simulink model "sim_accelerometersensor1"  (R2020b)
settings: Solver=FixedStepDiscrete  StartTime=0.0  StopTime=60  FixedStep=0.1  RelTol=1e-3  EnableMultiTasking=on
undefined symbols (not defined in the file): DiscIntNeverNeededParam
libraries: frdmk64flib x3, dspstat3 x2
settings Model: ExtModeTrigDuration=5  Creator=luca9  LastModifiedBy=luca9
settings OptimizationCC: EnhancedBackFolding=on  PassReuseOutputArgsAs=Individual arguments  ZeroExternalMemoryAtStartup=off  ZeroInternalMemoryAtStartup=off  MaxStackSize=64  OptimizeBlockOrder=speed  DifferentSizesBufferReuse=on  OptimizationCustomize=off  EfficientTunableParamExpr=on
settings DebuggingCC: ParameterTunabilityLossMsg=error
settings HardwareCC: ProdBitPerPointer=32  ProdBitPerSizeT=32  ProdBitPerPtrDiffT=32  ProdLargestAtomicInteger=Long  ProdLargestAtomicFloat=Double  ProdWordSize=32  ProdHWDeviceType=ARM Compatible->ARM Cortex
settings SFSimCC: MATLABDynamicMemAlloc=off
settings RTWCC: Description=Embedded Coder  SystemTargetFile=ert.tlc  HardwareBoard=NXP FRDM-K64F  TLCOptions="-aInlineSetEventsForThisBaseRateFcn=TLC_FALSE -aSuppressMultiTaskScheduler=TLC_FALSE  -aRateBasedStepFcn=0"  TemplateMakefile=ert_default_tmf  GenerateReport=on  Toolchain=GNU Tools for ARM Embedded Processors
settings CodeAppCC: ForceParamTrailComments=on  IgnoreCustomStorageClasses=off  OperatorAnnotations=on  SimulinkDataObjDesc=on  SFDataObjDesc=on  InsertBlockDesc=on

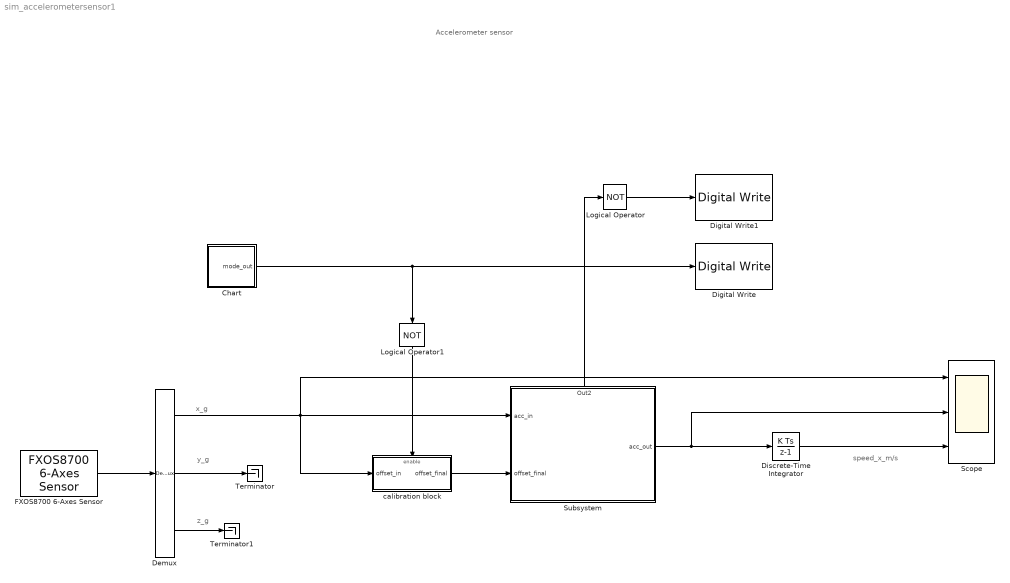
== system sim_accelerometersensor1 ==
  note: Accelerometer sensor
  note: speed_x_m/s
  note: z_g
  note: y_g
  note: x_g
  Chart : Stateflow chart  TreatAsAtomicUnit=on
  Demux : Demux  Outputs=3
  Digital Write : frdmk64flib/Digital Write  Whichpin=GREEN_LED
  Digital Write1 : frdmk64flib/Digital Write  Whichpin=RED_LED
  Discrete-Time Integrator : DiscreteIntegrator  SampleTime=-1  ICPrevOutput=DiscIntNeverNeededParam  ICPrevScaledInput=DiscIntNeverNeededParam
  FXOS8700 6-Axes Sensor : frdmk64flib/FXOS8700 6-Axes Sensor  Activesensor=Accelerometer only  ODR=50Hz  HybridODR=400Hz  Accelfullrange=-2g to +2g  SampleTime=-1
  Logical Operator : Logic  Operator=NOT  AllPortsSameDT=off  OutDataTypeStr=boolean
  Logical Operator1 : Logic  Operator=NOT  AllPortsSameDT=off  OutDataTypeStr=boolean
  Scope : Scope  NumInputPorts=3
  Subsystem : Subsystem
      settings: PortSchema="{\"entries\":[{\"content\":{\"sides\":[{\"content\":{\"connectorIds\":[\"In1\",\"In2\"]},\"type\":\"ConnectorPlacement.EquallySpacedRectSide\",\"uuid\":\"051b063d-3ab2-4142-9eb5-e7383778bf78\"},{\"content\":{\"connectorIds\":[\"Out1\"],\"side\":\"RIGHT\"},\"type\":\"ConnectorPlacement.EquallySpacedRectSide\",\"uuid\":\"8a890c9a-0c5b-4502-b4a6-1b5503535dea\"},{\"content\":{\"connectorIds\":[\"Out2\"],\"side\":\"TOP\"},\"type\":\"ConnectorPlacement.EquallySpacedRectSide\",\"uuid\":\"5543deee-079c-4823-8e07-12dd7eeba008\"}]},\"type\":\"ConnectorPlacement.EquallySpacedConnector\",\"uuid\":\"8e9d7cf8-ebda-403d-9c20-7172ebb8cffb\"}],\"packageUris\":[\"http://schema.mathworks.com/mf0/Connector/19700101\"],\"version\":\"1.0\"}"
  Terminator : Terminator
  Terminator1 : Terminator
  calibration block : Subsystem
  wires:
  FXOS8700 6-Axes Sensor/1 -> Demux/1
  Demux/2 -> Terminator/1
  Demux/3 -> Terminator1/1
  Subsystem/1(acc_out) -> Discrete-Time Integrator/1, Scope/2
  Chart/1(mode_out) -> Digital Write/1, Logical Operator1/1
  Demux/1 -> Subsystem/1(acc_in), calibration block/1(offset_in), Scope/1
  calibration block/1(offset_final) -> Subsystem/2(offset_final)
  Discrete-Time Integrator/1 -> Scope/3
  Logical Operator/1 -> Digital Write1/1
  Subsystem/2(Out2) -> Logical Operator/1
  Logical Operator1/1 -> calibration block/Enable

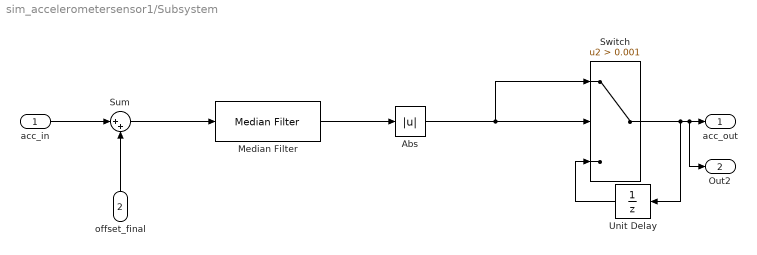
== system sim_accelerometersensor1/Subsystem ==
  acc_in : Inport
  offset_final : Inport  Port=2
  Abs : Abs
  Median Filter : dspstat3/Median Filter  WindowLength=5  SimulateUsing=Interpreted execution
      settings: SourceProductBaseCode=DS
  Sum : Sum  Inputs=|++
  Switch : Switch  Criteria=u2 > Threshold  Threshold=0.001
  Unit Delay : UnitDelay  SampleTime=-1  HasFrameUpgradeWarning=on
  acc_out : Outport
  Out2 : Outport  Port=2
  wires:
  Sum/1 -> Median Filter/1
  acc_in/1 -> Sum/1
  offset_final/1 -> Sum/2
  Median Filter/1 -> Abs/1
  Abs/1 -> Switch/2, Switch/1
  Unit Delay/1 -> Switch/3
  Switch/1 -> Unit Delay/1, Out2/1, acc_out/1

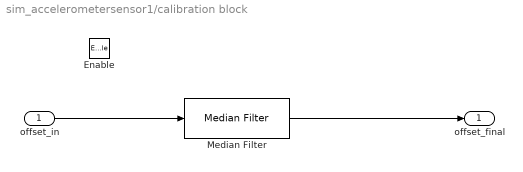
== system sim_accelerometersensor1/calibration block ==
  offset_in : Inport
  Enable : EnablePort
  Median Filter : dspstat3/Median Filter  WindowLength=128  SimulateUsing=Interpreted execution
      settings: SourceProductBaseCode=DS
  offset_final : Outport
  wires:
  Median Filter/1 -> offset_final/1
  offset_in/1 -> Median Filter/1

== stateflow chart sim_accelerometersensor1/Chart ==
  state calibration
    en:
    mode_out=0;
  state calibration1
    en:
    mode_out=1;
  (default) -> calibration
  calibration -> calibration1 : after(20,sec)
  data: mode_out output
